simulink model "motor_svpwm"  (R2022a)
settings: Solver=FixedStepDiscrete  StartTime=0.0  StopTime=2  FixedStep=1e-6  RelTol=1e-3
undefined symbols (not defined in the file or in its folder): DiscIntNeverNeededParam, TN, Udc
libraries: spsIGBTDiodeLib x4, spsGroundLib x3, spsDCVoltageSourceLib x2, spsDCMachineLib x1, simulink x1, spsVoltageMeasurementLib x1, spspowerguiLib x1
settings Model: Creator=57308  LastModifiedBy=57308
settings OptimizationCC: DefaultParameterBehavior=Inlined  UseDivisionForNetSlopeComputation=on  GainParamInheritBuiltInType=on  UseFloatMulNetSlope=on  InlineInvariantSignals=on  PassReuseOutputArgsAs=Individual arguments  ZeroExternalMemoryAtStartup=off  ZeroInternalMemoryAtStartup=off  NoFixptDivByZeroProtection=on  EfficientFloat2IntCast=on  LifeSpan=1  OptimizeBlockOrder=speed  DifferentSizesBufferReuse=on  EfficientTunableParamExpr=on
settings DebuggingCC: ParameterTunabilityLossMsg=error
settings HardwareCC: ProdBitPerPointer=32  ProdBitPerSizeT=32  ProdBitPerPtrDiffT=32  ProdLargestAtomicInteger=Long  ProdLargestAtomicFloat=Double  ProdWordSize=32  ProdLongLongMode=on  ProdHWDeviceType=NXP->Cortex-M4
settings SFSimCC: MATLABDynamicMemAlloc=off
settings RTWCC: SystemTargetFile=ert.tlc  GenCodeOnly=on  TemplateMakefile=ert_default_tmf  GenerateReport=on  LaunchReport=on
settings CodeAppCC: ForceParamTrailComments=on  IgnoreCustomStorageClasses=off  OperatorAnnotations=on  SimulinkDataObjDesc=on  SFDataObjDesc=on  CustomSymbolStrGlobalVar=rt$N$M  CustomSymbolStrType=$N$M  CustomSymbolStrFcn=$N$M$F  CustomSymbolStrMacro=$N$M  InsertBlockDesc=on
settings ERTTargetCC: TargetLangStandard=C99 (ISO)  IncludeMdlTerminateFcn=off  CombineSignalStateStructs=on  CodeInterfacePackaging=Reusable function  SupportComplex=off  SupportNonInlinedSFcns=on  InlinedParameterPlacement=NonHierarchical  ERTCustomFileTemplate=example_file_process.tlc  ERTFilePackagingFormat=CompactWithDataFile

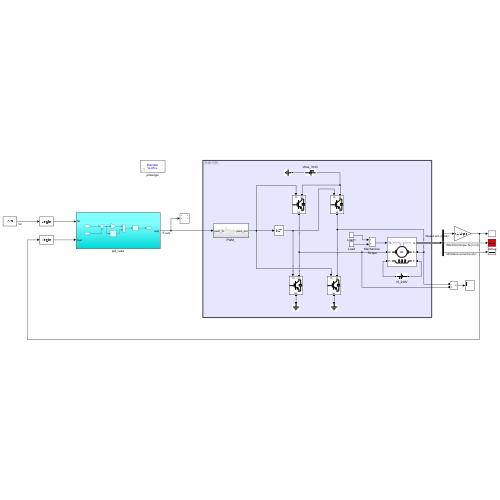
[thumbnail: Simulink's stored preview of the top-level diagram]
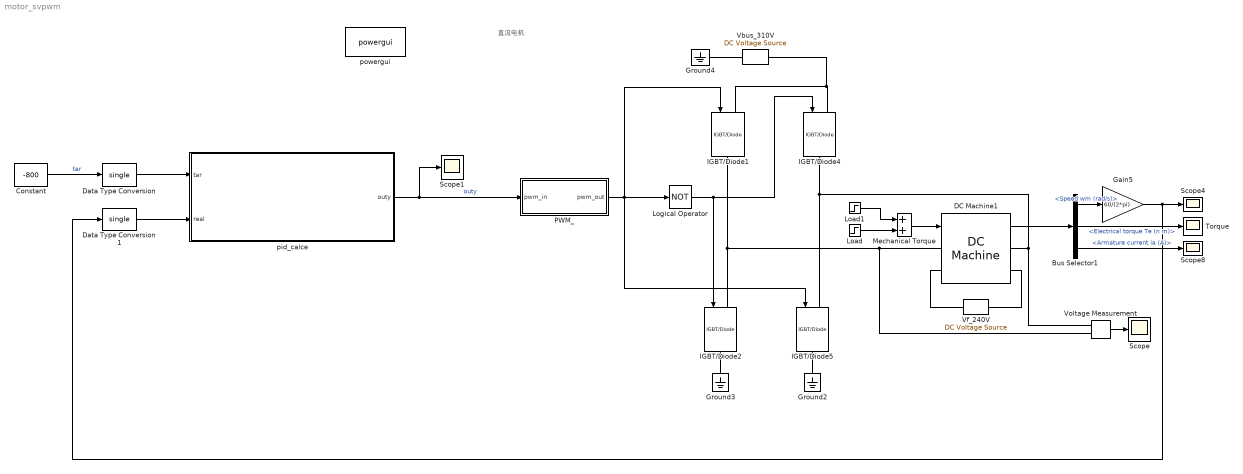
== system motor_svpwm ==
  note: 直流电机
  Bus Selector1 : BusSelector  OutputSignals=Speed wm (rad/s),Electrical torque Te (n m),Armature current ia (A)
  Constant : Constant  Value=-800
  DC Machine1 : spsDCMachineLib/DC Machine  PresetModel=No  MechanicalLoad=Torque TL  FieldType=Wound  ShowDetailedParameters=on  MeasurementBus=off  RLa="[ 0.6  0.012]"  RLf="[ 240  120]"  Laf=1.8  MachineConstant=Torque constant (N.m/A)  Ke=1.8  Kt=1.8  J=0.05  Bm=0  Tf=0  w0=0  Ifinit=1  TsPowergui=0  TsBlock=-1
  Data Type Conversion : DataTypeConversion  OutDataTypeStr=single  SaturateOnIntegerOverflow=off  RndMeth=Floor
  Data Type Conversion1 : DataTypeConversion  OutDataTypeStr=single  SaturateOnIntegerOverflow=off  RndMeth=Floor
  Gain5 : Gain  Gain=60/(2*pi)
  Ground2 : spsGroundLib/Ground  LConnTagsString=a
  Ground3 : spsGroundLib/Ground  LConnTagsString=a
  Ground4 : spsGroundLib/Ground  LConnTagsString=a
  IGBT/Diode{1..2,4..5} (4 alike) : spsIGBTDiodeLib/IGBT//Diode  Ron=1e-3  Rs=1e5  Cs=inf  Measurements=off
  Load : Step  Time=0.4  After=TN  SampleTime=0
  Load1 : Step  Time=0.6  After=-0.2*TN  SampleTime=0
  Logical Operator : Logic  Operator=NOT  AllPortsSameDT=off  OutDataTypeStr=boolean
  Mechanical Torque : Sum
  PWM_ : Subsystem
  Scope{,1,4,8} (4 alike) : Scope
  Torque : Scope
  Vbus_310V : spsDCVoltageSourceLib/DC Voltage Source  Amplitude=Udc  Measurements=None
  Vf_240V : spsDCVoltageSourceLib/DC Voltage Source  Amplitude=240  Measurements=None
  Voltage Measurement : spsVoltageMeasurementLib/Voltage Measurement  PhasorSimulation=off  OutputType=Complex  PSBequivalent=0
  pid_calce : Subsystem
  powergui : spspowerguiLib/powergui  Priority=1  SimulationMode=Discrete  SampleTime=1e-6  frequency=60  Iterations=50  frequencyindice=0  Pbase=100e6  ErrMax=1e-4  UnitsV=kV  UnitsW=MW  buscounter=0  FunctionMessages=off  echomessages=off  EnableUseOfTLC=off  CurrentSourceSwitches=off  DisableSnubberDevices=off  DisableRonSwitches=off  DisableVfSwitches=off  DisplayEquations=off  AutomaticDiscreteSolvers=off  SolverType=Tustin/Backward Euler (TBE)  Interpol=off  ExternalGateDelay=off  methode=off  Ts=100  x0status=blocks  SPID=on  SwTol=0  HookPort=off  NonlinearTolerance=1e-4  nMaxIteration=100  ContinueOnMaxIteration=off  RestoreLinks=warning  ResistiveCurrentMeasurement=off  Frange=[0:2:500]  Ylog=off  Xlog=on  ShowGrid=off  save=off  variable=ZData  structure=0  ZoomFFT=off  StartTime=0.0  cycles=1  DisplayStyle=1  fundamental=60  FreqAxis=off  MaxFrequency=1000  frequencyindicesteady=1  RmsSteady=1  display=off
  wires:
  pid_calce/1(outy) -> PWM_/1(pwm_in), Scope1/1  "outy"
  Constant/1 -> Data Type Conversion/1  "tar"
  Data Type Conversion/1 -> pid_calce/1(tar)
  Data Type Conversion1/1 -> pid_calce/2(real)
  Logical Operator/1 -> IGBT/Diode2/1, IGBT/Diode4/1
  Gain5/1 -> Scope4/1, Data Type Conversion1/1
  Bus Selector1/3 -> Scope8/1  "<Armature current ia (A)>"
  Bus Selector1/1 -> Gain5/1  "<Speed wm (rad/s)>"
  DC Machine1/1 -> Bus Selector1/1
  Load/1 -> Mechanical Torque/2
  Load1/1 -> Mechanical Torque/1
  PWM_/1(pwm_out) -> IGBT/Diode1/1, Logical Operator/1, IGBT/Diode5/1
  Voltage Measurement/1 -> Scope/1
  Bus Selector1/2 -> Torque/1  "<Electrical torque Te (n m)>"
  Mechanical Torque/1 -> DC Machine1/1
  connections:
  Vbus_310V/RConn1 -- IGBT/Diode4/LConn1 -- IGBT/Diode1/LConn1
  IGBT/Diode2/LConn1 -- DC Machine1/LConn1 -- Voltage Measurement/LConn1 -- IGBT/Diode1/RConn1
  IGBT/Diode5/LConn1 -- IGBT/Diode4/RConn1 -- Voltage Measurement/LConn2 -- DC Machine1/RConn1
  Vf_240V/RConn1 -- DC Machine1/LConn2
  Vbus_310V/LConn1 -- Ground4/LConn1
  Vf_240V/LConn1 -- DC Machine1/RConn2
  Ground2/LConn1 -- IGBT/Diode5/RConn1
  Ground3/LConn1 -- IGBT/Diode2/RConn1

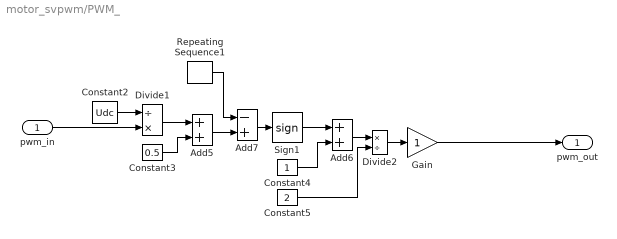
== system motor_svpwm/PWM_ ==
  pwm_in : Inport
  Add5 : Sum
  Add6 : Sum
  Add7 : Sum  Inputs=-+
  Constant2 : Constant  Value=Udc
  Constant3 : Constant  Value=0.5
  Constant4 : Constant
  Constant5 : Constant  Value=2
  Divide1 : Product  Inputs=/*
  Divide2 : Product  Inputs=*/
  Gain : Gain
  Repeating Sequence1 : simulink/Sources/Repeating Sequence  rep_seq_t=[0 100e-6 200e-6]  rep_seq_y=[0 1 0]
  Sign1 : Signum
  pwm_out : Outport
  wires:
  Repeating Sequence1/1 -> Add7/1
  pwm_in/1 -> Divide1/2
  Sign1/1 -> Add6/1
  Divide1/1 -> Add5/1
  Constant5/1 -> Divide2/2
  Constant2/1 -> Divide1/1
  Divide2/1 -> Gain/1
  Add7/1 -> Sign1/1
  Constant3/1 -> Add5/2
  Add5/1 -> Add7/2
  Constant4/1 -> Add6/2
  Add6/1 -> Divide2/1
  Gain/1 -> pwm_out/1

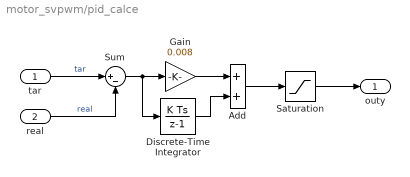
== system motor_svpwm/pid_calce ==
  tar : Inport  OutDataTypeStr=single
  real : Inport  Port=2  OutDataTypeStr=single
  Add : Sum
  Discrete-Time Integrator : DiscreteIntegrator  gainval=0.8  SampleTime=-1  UpperSaturationLimit=Udc  LowerSaturationLimit=-Udc  StateName=Integrator  ICPrevOutput=DiscIntNeverNeededParam  ICPrevScaledInput=DiscIntNeverNeededParam  StateMustResolveToSignalObject=on
  Gain : Gain  Gain=0.008  ParamDataTypeStr=single
  Saturation : Saturate  UpperLimit=Udc  LowerLimit=-Udc
  Sum : Sum  Inputs=|+-
  outy : Outport  OutDataTypeStr=single
  wires:
  real/1 -> Sum/2  "real"
  Gain/1 -> Add/1
  Add/1 -> Saturation/1
  tar/1 -> Sum/1  "tar"
  Sum/1 -> Gain/1, Discrete-Time Integrator/1
  Discrete-Time Integrator/1 -> Add/2
  Saturation/1 -> outy/1
